simulink model "k64f_rateadapt"  (R2020a)
settings: Solver=FixedStepAuto  StartTime=0.0  StopTime=1.0  FixedStep=1E-3  RelTol=1e-3  EnableMultiTasking=on
undefined symbols (not defined in the file): A0, A1, D0, D1, D10, D11, D12, D13, D2, D3, D4, D5, D6, D7, D8, D9, PTA0, PTA1, PTA2, PTB2, PTB23, PTB3, PTB9, PTC16, PTC17, PTC2, PTC3, PTC4, PTD0, PTD1, PTD2, PTD3
libraries: frdmk64flib x23, etargetslib x2
settings Model: ExtModeTrigDuration=5  Creator=Mostafa  LastModifiedBy=Kevin Chen
settings OptimizationCC: EnhancedBackFolding=on  PassReuseOutputArgsAs=Individual arguments  ZeroExternalMemoryAtStartup=off  ZeroInternalMemoryAtStartup=off  MaxStackSize=64  OptimizeBlockOrder=speed  DifferentSizesBufferReuse=on  OptimizationCustomize=off  EfficientTunableParamExpr=on
settings DebuggingCC: ParameterPrecisionLossMsg=none  ParameterTunabilityLossMsg=error
settings HardwareCC: ProdBitPerPointer=32  ProdBitPerSizeT=32  ProdBitPerPtrDiffT=32  ProdLargestAtomicInteger=Long  ProdLargestAtomicFloat=Double  ProdWordSize=32  ProdHWDeviceType=ARM Compatible->ARM Cortex  UseEmbeddedCoderFeatures=off
settings SFSimCC: MATLABDynamicMemAlloc=off
settings RTWCC: SystemTargetFile=ert.tlc  HardwareBoard=NXP FRDM-K64F  TemplateMakefile=ert_default_tmf  Toolchain=GNU Tools for ARM Embedded Processors
settings CodeAppCC: ForceParamTrailComments=on  IgnoreCustomStorageClasses=off  OperatorAnnotations=on  SimulinkDataObjDesc=on  SFDataObjDesc=on  InsertBlockDesc=on
settings ERTTargetCC: SupportNonInlinedSFcns=on

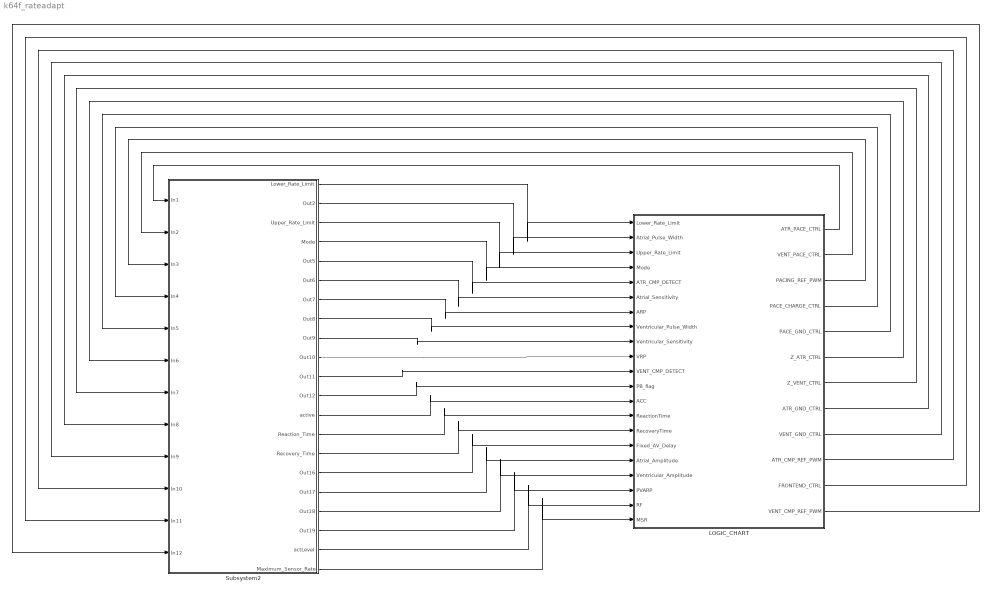
== system k64f_rateadapt ==
  LOGIC_CHART : Stateflow chart  TreatAsAtomicUnit=on
      settings: PortSchema="{\"entries\":[{\"content\":{\"sides\":[{\"content\":{\"connectorIds\":[\"In1\",\"In2\",\"In3\",\"In4\",\"In5\",\"In6\",\"In7\",\"In8\",\"In9\",\"In10\",\"In11\",\"In12\",\"In13\",\"In14\",\"In17\",\"In18\",\"In19\",\"In20\",\"In21\",\"In15\",\"In16\"]},\"type\":\"ConnectorPlacement.EquallySpacedRectSide\",\"uuid\":\"2532a15d-7e3f-497c-8f71-038aa275bfb3\"},{\"content\":{\"connectorIds\":[\"Out1\",\"Out2\",\"Out3\",\"Out4\",\"Out5\",\"Out6\",\"Out7\",\"Out8\",\"Out9\",\"Out10\",\"Out11\",\"Out12\"],\"side\":\"RIGHT\"},\"type\":\"ConnectorPlacement.EquallySpacedRectSide\",\"uuid\":\"b4365400-6566-41c9-a565-c69f74d7ec16\"},{\"content\":{\"connectorIds\":[],\"side\":\"TOP\"},\"type\":\"ConnectorPlacement.EquallySpacedRectSide\",\"uuid\":\"ee6cfb42-5307-4b65-a86e-84b69df89ddc\"}]},\"type\":\"ConnectorPlacement.EquallySpacedConnector\",\"uuid\":\"ec232628-3749-49a9-9e57-0299de21913c\"}],\"packageUris\":[\"http://schema.mathworks.com/mf0/Connector/19700101\"],\"version\":\"1.0\"}"
  Subsystem2 : Subsystem
  wires:
  LOGIC_CHART/1(ATR_PACE_CTRL) -> Subsystem2/1(In1)
  LOGIC_CHART/2(VENT_PACE_CTRL) -> Subsystem2/2(In2)
  LOGIC_CHART/3(PACING_REF_PWM) -> Subsystem2/3(In3)
  LOGIC_CHART/4(PACE_CHARGE_CTRL) -> Subsystem2/4(In4)
  LOGIC_CHART/5(PACE_GND_CTRL) -> Subsystem2/5(In5)
  LOGIC_CHART/6(Z_ATR_CTRL) -> Subsystem2/6(In6)
  LOGIC_CHART/7(Z_VENT_CTRL) -> Subsystem2/7(In7)
  LOGIC_CHART/8(ATR_GND_CTRL) -> Subsystem2/8(In8)
  LOGIC_CHART/9(VENT_GND_CTRL) -> Subsystem2/9(In9)
  LOGIC_CHART/10(ATR_CMP_REF_PWM) -> Subsystem2/10(In10)
  LOGIC_CHART/11(FRONTEND_CTRL) -> Subsystem2/11(In11)
  LOGIC_CHART/12(VENT_CMP_REF_PWM) -> Subsystem2/12(In12)
  Subsystem2/1(Lower_Rate_Limit) -> LOGIC_CHART/1(Lower_Rate_Limit)
  Subsystem2/2(Out2) -> LOGIC_CHART/2(Atrial_Pulse_Width)
  Subsystem2/3(Upper_Rate_Limit) -> LOGIC_CHART/3(Upper_Rate_Limit)
  Subsystem2/4(Mode) -> LOGIC_CHART/4(Mode)
  Subsystem2/5(Out5) -> LOGIC_CHART/5(ATR_CMP_DETECT)
  Subsystem2/6(Out6) -> LOGIC_CHART/6(Atrial_Sensitivity)
  Subsystem2/7(Out7) -> LOGIC_CHART/7(ARP)
  Subsystem2/8(Out8) -> LOGIC_CHART/8(Ventricular_Pulse_Width)
  Subsystem2/9(Out9) -> LOGIC_CHART/9(Ventricular_Sensitivity)
  Subsystem2/10(Out10) -> LOGIC_CHART/10(VRP)
  Subsystem2/11(Out11) -> LOGIC_CHART/11(VENT_CMP_DETECT)
  Subsystem2/12(Out12) -> LOGIC_CHART/12(PB_flag)
  Subsystem2/13(active) -> LOGIC_CHART/13(ACC)
  Subsystem2/14(Reaction_Time) -> LOGIC_CHART/14(ReactionTime)
  Subsystem2/15(Recovery_Time) -> LOGIC_CHART/17(RecoveryTime)
  Subsystem2/16(Out16) -> LOGIC_CHART/18(Fixed_AV_Delay)
  Subsystem2/17(Out17) -> LOGIC_CHART/19(Atrial_Amplitude)
  Subsystem2/18(Out18) -> LOGIC_CHART/20(Ventricular_Amplitude)
  Subsystem2/19(Out19) -> LOGIC_CHART/21(PVARP)
  Subsystem2/20(actLevel) -> LOGIC_CHART/15(RF)
  Subsystem2/21(Maximum_Sensor_Rate) -> LOGIC_CHART/16(MSR)

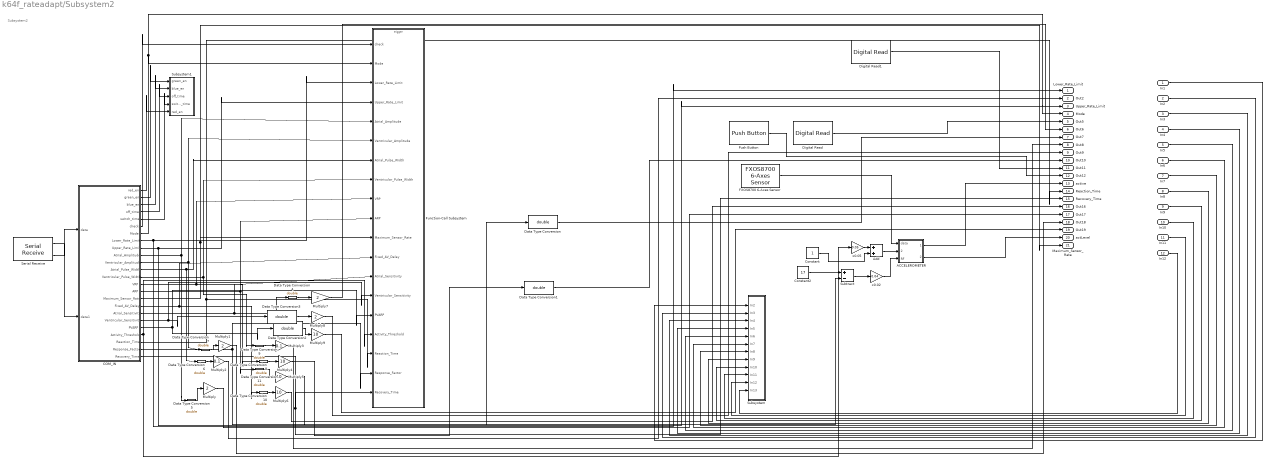
== system k64f_rateadapt/Subsystem2 ==
  note: Subsystem2
  In1 : Inport
  In2 : Inport  Port=2
  In3 : Inport  Port=3
  In4 : Inport  Port=4
  In5 : Inport  Port=5
  In6 : Inport  Port=6
  In7 : Inport  Port=7
  In8 : Inport  Port=8
  In9 : Inport  Port=9
  In10 : Inport  Port=10
  In11 : Inport  Port=11
  In12 : Inport  Port=12
  ACCELEROMETER : Stateflow chart  TreatAsAtomicUnit=on
  Add : Sum
  COM_IN : Stateflow chart  TreatAsAtomicUnit=on
      settings: PortSchema="{\"entries\":[{\"content\":{\"sides\":[{\"content\":{\"connectorIds\":[\"In1\",\"In2\"]},\"type\":\"ConnectorPlacement.EquallySpacedRectSide\",\"uuid\":\"0622ed0d-a63c-4425-81a9-1b700e3d40e7\"},{\"content\":{\"connectorIds\":[\"Out1\",\"Out2\",\"Out3\",\"Out4\",\"Out5\",\"Out24\",\"Out6\",\"Out7\",\"Out8\",\"Out9\",\"Out10\",\"Out11\",\"Out12\",\"Out13\",\"Out14\",\"Out15\",\"Out16\",\"Out17\",\"Out18\",\"Out19\",\"Out20\",\"Out21\",\"Out22\",\"Out23\"],\"side\":\"RIGHT\"},\"type\":\"ConnectorPlacement.EquallySpacedRectSide\",\"uuid\":\"1b9db426-091c-4aed-ac90-de166372e318\"},{\"content\":{\"connectorIds\":[],\"side\":\"TOP\"},\"type\":\"ConnectorPlacement.EquallySpacedRectSide\",\"uuid\":\"c8726b50-1e98-4bba-9c0e-57637e7ead5e\"}]},\"type\":\"ConnectorPlacement.EquallySpacedConnector\",\"uuid\":\"eab4333c-b3ae-429b-bd5d-289e8cbf8e60\"}],\"packageUris\":[\"http://schema.mathworks.com/mf0/Connector/19700101\"],\"version\":\"1.0\"}"
  Constant : Constant
  Constant2 : Constant  Value=17
  Data Type Conversion{,1..11} (12 alike) : DataTypeConversion  OutDataTypeStr=double
  Digital Read : frdmk64flib/Digital Read  Whichpin=PTC16 (D0)  SampleTime=-1
  Digital Read1 : frdmk64flib/Digital Read  Whichpin=PTC17 (D1)  SampleTime=-1
  FXOS8700 6-Axes Sensor : frdmk64flib/FXOS8700 6-Axes Sensor  Activesensor=Accelerometer only  ODR=800Hz  HybridODR=400Hz  Accelfullrange=-4g to +4g  SampleTime=-1
  Function-Call Subsystem : Subsystem  TreatAsAtomicUnit=on
  Multiply{,1,7..8} (4 alike) : Gain  Gain=2
  Multiply2 : Gain  Gain=0.1
  Multiply3 : Gain  Gain=0.1
  Multiply{4..6,9} (4 alike) : Gain  Gain=10
  Push Button : frdmk64flib/Push Button  Whichswitch=SW2  SampleTime1=-1
  Serial Receive : frdmk64flib/Serial Receive  SCIModule=0  Baudrate=uint32(9600)  Parity=None  StopBits=1  HardwareFlowControl=None  ByteOrder=LittleEndian  DataType=uint8  DataLength=20  BlockingMode=off  OutputStatus=on  SampleTime=-1
  Subsystem : Subsystem
  Subsystem1 : Subsystem
  Subtract : Sum  Inputs=+-
  x0.02 : Gain  Gain=0.04
  x0.05 : Gain  Gain=0.05
  Lower_Rate_Limit : Outport
  Out2 : Outport  Port=2
  Upper_Rate_Limit : Outport  Port=3
  Mode : Outport  Port=4
  Out5 : Outport  Port=5
  Out6 : Outport  Port=6
  Out7 : Outport  Port=7
  Out8 : Outport  Port=8
  Out9 : Outport  Port=9
  Out10 : Outport  Port=10
  Out11 : Outport  Port=11
  Out12 : Outport  Port=12
  active : Outport  Port=13
  Reaction_Time : Outport  Port=14
  Recovery_Time : Outport  Port=15
  Out16 : Outport  Port=16
  Out17 : Outport  Port=17
  Out18 : Outport  Port=18
  Out19 : Outport  Port=19
  actLevel : Outport  Port=20
  Maximum_Sensor_Rate : Outport  Port=21
  wires:
  Data Type Conversion5/1 -> Multiply/1
  In11/1 -> Subsystem/11(In12)
  COM_IN/2(green_en) -> Subsystem1/1(green_en)
  FXOS8700 6-Axes Sensor/1 -> ACCELEROMETER/1(data)
  ACCELEROMETER/1(active) -> active/1
  COM_IN/10(Ventricular_Amplitude) -> Data Type Conversion7/1, Function-Call Subsystem/6(Ventricular_Amplitude)
  COM_IN/7(Lower_Rate_Limit) -> Lower_Rate_Limit/1, Function-Call Subsystem/3(Lower_Rate_Limit)
  x0.02/1 -> ACCELEROMETER/3(RF)
  COM_IN/20(Activity_Threshold) -> x0.05/1, Function-Call Subsystem/16(Activity_Threshold)
  Data Type Conversion9/1 -> Multiply3/1
  Serial Receive/1 -> COM_IN/2(data1)
  COM_IN/12(Ventricular_Pulse_Width) -> Data Type Conversion9/1, Function-Call Subsystem/8(Ventricular_Pulse_Width)
  COM_IN/11(Atrial_Pulse_Width) -> Function-Call Subsystem/7(Atrial_Pulse_Width), Data Type Conversion6/1
  Add/1 -> ACCELEROMETER/2(Threshold)
  Data Type Conversion4/1 -> Multiply7/1
  COM_IN/18(Ventricular_Sensitivity) -> Data Type Conversion3/1, Function-Call Subsystem/14(Ventricular_Sensitivity)
  COM_IN/17(Atrial_Sensitivity) -> Data Type Conversion4/1, Function-Call Subsystem/13(Atrial_Sensitivity)
  COM_IN/15(Maximum_Sensor_Rate) -> Maximum_Sensor_Rate/1, Function-Call Subsystem/11(Maximum_Sensor_Rate)
  COM_IN/16(Fixed_AV_Delay) -> Data Type Conversion10/1, Function-Call Subsystem/12(Fixed_AV_Delay)
  COM_IN/6(Mode) -> Mode/1, Function-Call Subsystem/2(Mode)
  Data Type Conversion2/1 -> Multiply9/1
  In4/1 -> Subsystem/4(In5)
  Data Type Conversion3/1 -> Multiply8/1
  Data Type Conversion/1 -> Out7/1
  Data Type Conversion7/1 -> Multiply1/1
  In8/1 -> Subsystem/8(In9)
  Data Type Conversion11/1 -> Multiply5/1
  In6/1 -> Subsystem/6(In7)
  Multiply1/1 -> Out18/1
  COM_IN/21(Reaction_Time) -> Reaction_Time/1, Function-Call Subsystem/17(Reaction_Time)
  Multiply9/1 -> Out19/1
  x0.05/1 -> Add/1
  Constant2/1 -> Subtract/1
  In1/1 -> Subsystem/1(In2)
  Constant/1 -> Add/2
  COM_IN/4(off_time) -> Subsystem1/3(off_time)
  In7/1 -> Subsystem/7(In8)
  COM_IN/9(Atrial_Amplitude) -> Data Type Conversion5/1, Function-Call Subsystem/5(Atrial_Amplitude)
  Data Type Conversion10/1 -> Multiply6/1
  Subtract/1 -> x0.02/1
  COM_IN/13(VRP) -> Data Type Conversion8/1, Function-Call Subsystem/9(VRP)
  Data Type Conversion1/1 -> Out10/1
  COM_IN/19(PVARP) -> Data Type Conversion2/1, Function-Call Subsystem/15(PVARP)
  COM_IN/8(Upper_Rate_Limit) -> Upper_Rate_Limit/1, Function-Call Subsystem/4(Upper_Rate_Limit)
  COM_IN/24(check) -> Function-Call Subsystem/1(check)
  COM_IN/22(Response_Factor) -> Subtract/2, Function-Call Subsystem/18(Response_Factor)
  Digital Read1/1 -> Out11/1
  COM_IN/23(Recovery_Time) -> Recovery_Time/1, Function-Call Subsystem/19(Recovery_Time)
  COM_IN/14(ARP) -> Data Type Conversion11/1, Function-Call Subsystem/10(ARP)
  Data Type Conversion6/1 -> Multiply2/1
  Push Button/1 -> Out12/1
  Multiply4/1 -> Data Type Conversion1/1
  Serial Receive/2 -> COM_IN/1(data)
  COM_IN/5(switch_time) -> Subsystem1/4(switch_time)
  In2/1 -> Subsystem/2(In3)
  COM_IN/3(blue_en) -> Subsystem1/2(blue_en)
  COM_IN/1(red_en) -> Subsystem1/5(red_en)
  Multiply5/1 -> Data Type Conversion/1
  ACCELEROMETER/2(actLevel) -> actLevel/1
  Data Type Conversion8/1 -> Multiply4/1
  In3/1 -> Subsystem/3(In4)
  In9/1 -> Subsystem/9(In10)
  Digital Read/1 -> Out5/1
  In5/1 -> Subsystem/5(In6)
  In12/1 -> Subsystem/12(In13)
  In10/1 -> Subsystem/10(In11)
  Multiply7/1 -> Out6/1
  Multiply6/1 -> Out16/1
  Multiply8/1 -> Out9/1
  Multiply2/1 -> Out2/1
  Multiply3/1 -> Out8/1
  Multiply/1 -> Out17/1

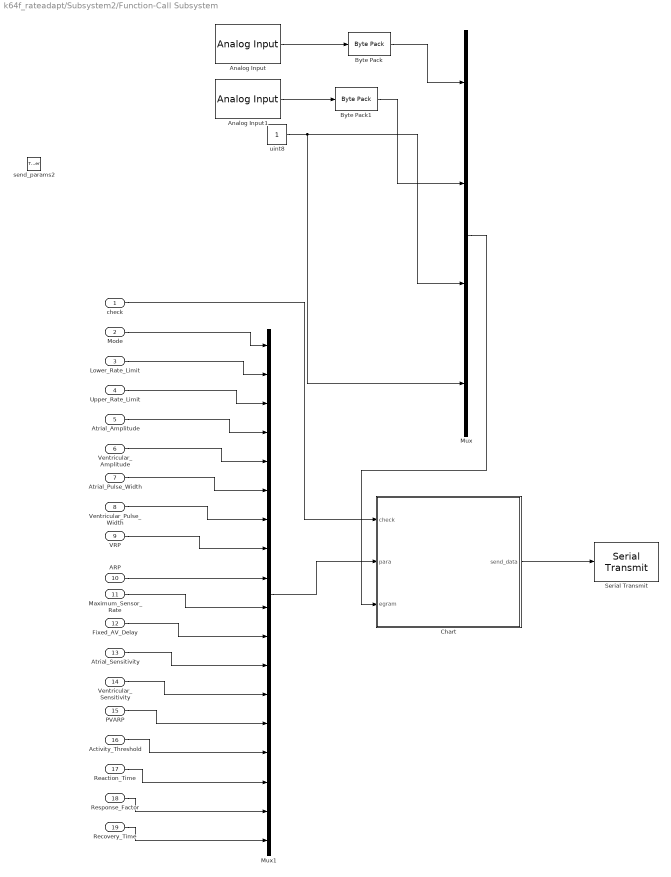
== system k64f_rateadapt/Subsystem2/Function-Call Subsystem ==
  check : Inport
  Mode : Inport  Port=2
  Lower_Rate_Limit : Inport  Port=3
  Upper_Rate_Limit : Inport  Port=4
  Atrial_Amplitude : Inport  Port=5
  Ventricular_Amplitude : Inport  Port=6
  Atrial_Pulse_Width : Inport  Port=7
  Ventricular_Pulse_Width : Inport  Port=8
  VRP : Inport  Port=9
  ARP : Inport  Port=10
  Maximum_Sensor_Rate : Inport  Port=11
  Fixed_AV_Delay : Inport  Port=12
  Atrial_Sensitivity : Inport  Port=13
  Ventricular_Sensitivity : Inport  Port=14
  PVARP : Inport  Port=15
  Activity_Threshold : Inport  Port=16
  Reaction_Time : Inport  Port=17
  Response_Factor : Inport  Port=18
  Recovery_Time : Inport  Port=19
  send_params2 : TriggerPort  TriggerType=function-call  IsSimulinkFunction=on  FunctionName=send_params2  VariantControl=Variant
  Analog Input : frdmk64flib/Analog Input  Whichpin=PTB2 (A0)  SampleTime=-1
  Analog Input1 : frdmk64flib/Analog Input  Whichpin=PTB3 (A1)  SampleTime=-1
  Byte Pack : etargetslib/Byte Pack  datatypes={'double'}  byteAlign=1
  Byte Pack1 : etargetslib/Byte Pack  datatypes={'double'}  byteAlign=1
  Chart : Stateflow chart  TreatAsAtomicUnit=on
  Mux : Mux
  Mux1 : Mux  Inputs=18
  Serial Transmit : frdmk64flib/Serial Transmit  SCIModule=0  Baudrate=uint32(9600)  Parity=None  StopBits=1  HardwareFlowControl=None  ByteOrder=LittleEndian  BlockingMode=on  OutputStatus=off
  uint8 : Constant  OutDataTypeStr=uint8
  wires:
  Mode/1 -> Mux1/1
  check/1 -> Chart/1(check)
  Analog Input1/1 -> Byte Pack1/1
  Chart/1(send_data) -> Serial Transmit/1
  Lower_Rate_Limit/1 -> Mux1/2
  Mux1/1 -> Chart/2(para)
  Upper_Rate_Limit/1 -> Mux1/3
  Mux/1 -> Chart/3(egram)
  Atrial_Amplitude/1 -> Mux1/4
  uint8/1 -> Mux/4, Mux/3
  Analog Input/1 -> Byte Pack/1
  Byte Pack/1 -> Mux/1
  Byte Pack1/1 -> Mux/2
  Ventricular_Amplitude/1 -> Mux1/5
  Atrial_Pulse_Width/1 -> Mux1/6
  Ventricular_Pulse_Width/1 -> Mux1/7
  VRP/1 -> Mux1/8
  Maximum_Sensor_Rate/1 -> Mux1/10
  Fixed_AV_Delay/1 -> Mux1/11
  Atrial_Sensitivity/1 -> Mux1/12
  Ventricular_Sensitivity/1 -> Mux1/13
  PVARP/1 -> Mux1/14
  Reaction_Time/1 -> Mux1/16
  Activity_Threshold/1 -> Mux1/15
  Response_Factor/1 -> Mux1/17
  Recovery_Time/1 -> Mux1/18
  ARP/1 -> Mux1/9

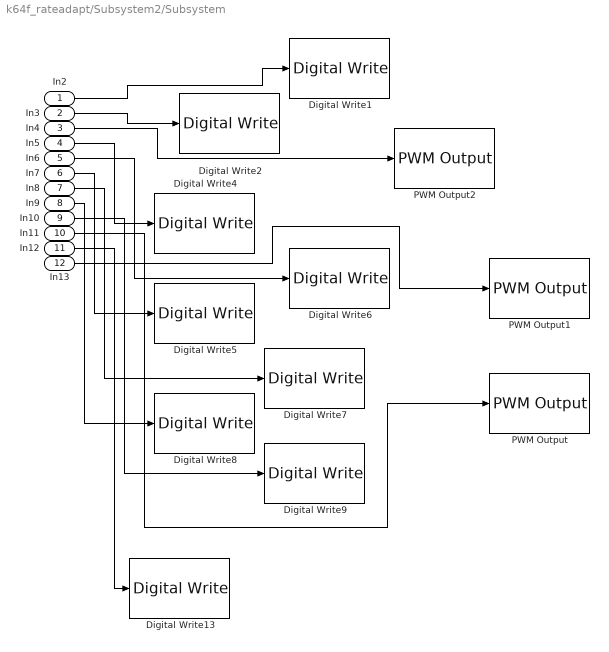
== system k64f_rateadapt/Subsystem2/Subsystem ==
  In2 : Inport
  In3 : Inport  Port=2
  In4 : Inport  Port=3
  In5 : Inport  Port=4
  In6 : Inport  Port=5
  In7 : Inport  Port=6
  In8 : Inport  Port=7
  In9 : Inport  Port=8
  In10 : Inport  Port=9
  In11 : Inport  Port=10
  In12 : Inport  Port=11
  In13 : Inport  Port=12
  Digital Write1 : frdmk64flib/Digital Write  Whichpin=PTA0 (D8)
  Digital Write13 : frdmk64flib/Digital Write  Whichpin=PTD1 (D13)
  Digital Write2 : frdmk64flib/Digital Write  Whichpin=PTC4 (D9)
  Digital Write4 : frdmk64flib/Digital Write  Whichpin=PTB9 (D2)
  Digital Write5 : frdmk64flib/Digital Write  Whichpin=PTB23 (D4)
  Digital Write6 : frdmk64flib/Digital Write  Whichpin=PTD0 (D10)
  Digital Write7 : frdmk64flib/Digital Write  Whichpin=PTC3 (D7)
  Digital Write8 : frdmk64flib/Digital Write  Whichpin=PTD2 (D11)
  Digital Write9 : frdmk64flib/Digital Write  Whichpin=PTD3 (D12)
  PWM Output : frdmk64flib/PWM Output  Whichpin=PTC2 (D6)  InitialFrequency=2000  InitialDutyCycle=100
  PWM Output1 : frdmk64flib/PWM Output  Whichpin=PTA1 (D3)  InitialFrequency=2000  InitialDutyCycle=0
  PWM Output2 : frdmk64flib/PWM Output  Whichpin=PTA2 (D5)  InitialFrequency=2000  InitialDutyCycle=100
  wires:
  In5/1 -> Digital Write4/1
  In9/1 -> Digital Write8/1
  In7/1 -> Digital Write5/1
  In3/1 -> Digital Write2/1
  In6/1 -> Digital Write6/1
  In4/1 -> PWM Output2/1
  In8/1 -> Digital Write7/1
  In10/1 -> Digital Write9/1
  In2/1 -> Digital Write1/1
  In12/1 -> Digital Write13/1
  In11/1 -> PWM Output/1
  In13/1 -> PWM Output1/1

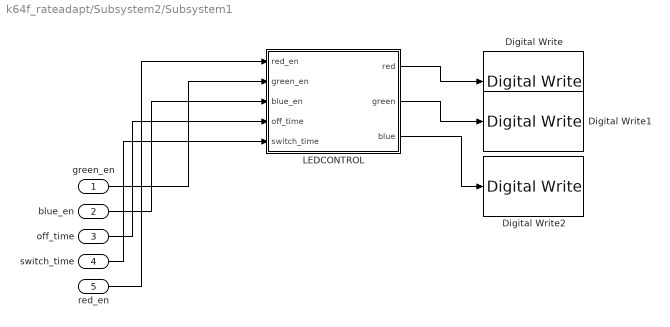
== system k64f_rateadapt/Subsystem2/Subsystem1 ==
  green_en : Inport
  blue_en : Inport  Port=2
  off_time : Inport  Port=3
  switch_time : Inport  Port=4
  red_en : Inport  Port=5
  Digital Write : frdmk64flib/Digital Write  Whichpin=RED_LED
  Digital Write1 : frdmk64flib/Digital Write  Whichpin=GREEN_LED
  Digital Write2 : frdmk64flib/Digital Write  Whichpin=BLUE_LED
  LEDCONTROL : Stateflow chart  TreatAsAtomicUnit=on
  wires:
  LEDCONTROL/1(red) -> Digital Write/1
  green_en/1 -> LEDCONTROL/2(green_en)
  LEDCONTROL/3(blue) -> Digital Write2/1
  switch_time/1 -> LEDCONTROL/5(switch_time)
  LEDCONTROL/2(green) -> Digital Write1/1
  red_en/1 -> LEDCONTROL/1(red_en)
  blue_en/1 -> LEDCONTROL/3(blue_en)
  off_time/1 -> LEDCONTROL/4(off_time)

== stateflow chart k64f_rateadapt/Subsystem2/COM_IN ==
  settings: executeAtInitialization=1
  state AOO
    entry:
    Mode=data1(3);
    Lower_Rate_Limit = data1(4);
    Upper_Rate_Limit = data1(5);
    Atrial_Amplitude = data1(6);
    Ventricular_Amplitude =data1(7);
    Atrial_Pulse_Width = data1(8);
    Ventricular_Pulse_Width = data1(9);
    VRP = data1(10);
    ARP = data1(11);
    Maximum_Sensor_Rate = data1(12);
    Fixed_AV_Delay = data1(13);
    Atrial_Sensitivity = data1(14);
    Ventricular_Sensitivity =data1(15);
    PVARP = data1(16);
    Activity_Threshold = data1(17);
    Reaction_Time = data1(18);
    Response_Factor = data1(19);
    Recovery_Time = data1(20);
    blue_en=0;
    red_en=0;
    green_en=1;
  state Idle
    entry:
    red_en=1;
    green_en=0;
    blue_en=0;
    off_time=0.5;
    switch_time=200;
  state Standby
    entry:
    red_en=0;
    blue_en=1;
    green_en=0;
    check=0;
  state ECHO_PARAM
    entry:
    check=49;
    send_params2();
    blue_en=0;
    red_en=1;
  state ECHO_EGRAM
    entry:
    check=47;
    send_params2();
    blue_en=1;
    green_en=1;
  (default) -> Idle
  AOO -> Standby : [after(2,sec)]
  (junction 205) -> AOO [order 1] : [data1(2)==hex2dec("55")]
  Idle -> Standby
  (junction 205) -> ECHO_EGRAM [order 3] : [data1(2)==hex2dec("47")]
  (junction 214) -> (junction 205) : [data1(1)==hex2dec("16")]
  (junction 205) -> ECHO_PARAM [order 2] : [data1(2)==hex2dec("49")]
  ECHO_EGRAM -> Standby [order 1] : [data1(2)==hex2dec("62")]
  Standby -> (junction 214) : [data==0]
  ECHO_PARAM -> Standby : [after(2,sec)]
  ECHO_EGRAM -> ECHO_EGRAM [order 2] : [after(1,msec)]
  data: data input uint8; data1 input uint8; red_en output uint8; green_en output uint8; blue_en output 'uint8'; off_time output 'single'; switch_time output 'uint16'; Mode output; Lower_Rate_Limit output; Upper_Rate_Limit output; Atrial_Amplitude output; Ventricular_Amplitude output; Atrial_Pulse_Width output; Ventricular_Pulse_Width output; VRP output; ARP output; Maximum_Sensor_Rate output; Fixed_AV_Delay output; Atrial_Sensitivity output; Ventricular_Sensitivity output; PVARP output; Activity_Threshold output; Reaction_Time output; Response_Factor output; Recovery_Time output; check output

== stateflow chart k64f_rateadapt/Subsystem2/ACCELEROMETER ==
  state Enter
    entry:
    active=0;
    actLevel=0;
  state Ini
    entry:
    Timing=0;
    acc=0;
  state H
    entry:
    acc=acc+norm(data);
    %update the motion level every 0.5s
    if(Timing==500)
    acc=acc/100; %taking average of acc over 0.5s
    if(acc>Threshold)
    active=1;
    if((acc-Threshold)>=RF)
    actLevel=100; %MSR will be reached if actLevel=100
    else
    %actLevel is the proportion of acc above threshold, in percentage
    actLevel=(acc-Threshold)/RF*100;
    end
    else %if acc is below threshold
    active=0;
    actLevel=0;
    end
    end
  (default) -> Enter
  Enter -> Ini
  Ini -> H
  H -> Ini [order 2] : [Timing>=500]
  H -> H [order 1] : [after(5,msec)&&Timing<500]{Timing=Timing+5}
      | %accumulate new motion data every 5ms
  data: data input; active output; actLevel output; acc local; Timing local; Threshold input; RF input

== stateflow chart k64f_rateadapt/LOGIC_CHART ==
  state VOO_CHARGING
    entry:
    %parameters for charging c22
    ATR_PACE_CTRL= false;
    VENT_PACE_CTRL = false;
    PACING_REF_PWM = Ventricular_Amplitude;
    PACE_CHARGE_CTRL = true;
    %parameters for discharging into c11
    PACE_GND_CTRL = true;
    VENT_PACE_CTRL = false;
    Z_ATR_CTRL = false;
    Z_VENT_CTRL = false;
    ATR_PACE_CTRL= false;
    ATR_GND_CTRL = false;
    VENT_GND_CTRL = true;
    if(Mode==9) %if it's rate adaptive
    if(ACC==1) %if activity above threshold
    %if rate is lower than the expected rate at the detected activity level
    %RF is the actLevel from Accelerometer FSM, which
    % is the proportion of acc above threshold, in percentage
    if((Rate-Lower_Rate_Limit)<((MSR-Lower_Rate_Limit)*RF/100))
    %increase Rate at the rate required to reach MSR from LRL within reaction time
    Rate=(Rate+(MSR-Lower_Rate_Limit)/ReactionTime*60/Rate);
    else
    %rate stays at the expected rate, determined from the current MSR, LRL and RF
    Rate=((MSR-Lower_Rate_Limit)*RF/100+Lower_Rate_Limit);
    end
    else %Acc==0, below threshold
    if(Rate>Lower_Rate_Limit)
    %decrease Rate at the rate required to reach MSR from LRL within recovery time
    Rate=(Rate-(MSR-Lower_Rate_Limit)/RecoveryTime*60/Rate);
    else
    Rate=Lower_Rate_Limit;
    end
    end
    end
  state DELAY_STATE3
    %delay for bonus
  state VOO_PACING
    entry:
    PACE_CHARGE_CTRL = false;
    PACE_GND_CTRL = true;
    ATR_PACE_CTRL= false;
    ATR_GND_CTRL = false;
    Z_ATR_CTRL = false;
    Z_VENT_CTRL = false;
    VENT_GND_CTRL = false;
    VENT_PACE_CTRL = true;
  state DELAY_STATE
    %delay for bonus
  state AOO_CHARGING
    entry:
    %parameters for charging c22
    ATR_PACE_CTRL= false;
    VENT_PACE_CTRL = false;
    PACING_REF_PWM =  Atrial_Amplitude;
    PACE_CHARGE_CTRL = true;
    %parameters for discharging into c11
    PACE_GND_CTRL = true;
    VENT_PACE_CTRL = false;
    Z_ATR_CTRL = false;
    Z_VENT_CTRL = false;
    ATR_PACE_CTRL= false;
    ATR_GND_CTRL = true;
    VENT_GND_CTRL = false;
    if(Mode==7) %if it's rate adaptive
    %for detailed comments of the following part of code, refer to VOO(R) mode
    if(ACC==1)
    if((Rate-Lower_Rate_Limit)<((MSR-Lower_Rate_Limit)*RF/100))
    Rate=(Rate+(MSR-Lower_Rate_Limit)/ReactionTime*60/Rate);
    else
    Rate=((MSR-Lower_Rate_Limit)*RF/100+Lower_Rate_Limit);
    end
    else
    if(Rate>Lower_Rate_Limit)
    Rate=(Rate-(MSR-Lower_Rate_Limit)/RecoveryTime*60/Rate);
    else
    Rate=Lower_Rate_Limit;
    end
    end
    end
  state AOO_PACING
    entry:
    PACE_CHARGE_CTRL = false;
    PACE_GND_CTRL = true;
    ATR_PACE_CTRL= true;
    ATR_GND_CTRL = false;
    Z_ATR_CTRL = false;
    Z_VENT_CTRL = false;
    VENT_GND_CTRL = false;
    VENT_PACE_CTRL = false;
  state Initial
    entry:
    delay=0;
    Rate=Lower_Rate_Limit;
    %delay is used in AAI(R)&VVI(R)
    %to correct for delay caused
    %by ARP and VRP
    %Rate is fixed to LRL if it's not in rate adaptive
    %modes, and it's changeable
    %if used in rate adaptive modes
  state AAI_CHARGING
    entry:
    %parameters for charging c22
    ATR_PACE_CTRL= false;
    VENT_PACE_CTRL = false;
    PACING_REF_PWM =  Atrial_Amplitude;
    PACE_CHARGE_CTRL = true;
    %parameters for discharging into c11
    PACE_GND_CTRL = true;
    VENT_PACE_CTRL = false;
    Z_ATR_CTRL = false;
    Z_VENT_CTRL = false;
    ATR_PACE_CTRL= false;
    ATR_GND_CTRL = true;
    VENT_GND_CTRL = false;
    %parameters for sensing
    ATR_CMP_REF_PWM=Atrial_Sensitivity;
    FRONTEND_CTRL= true;
    %timing for an expected natural heart event
    Timing=int16(0);
    if(Mode==8) %if it's rate adaptive
    %for detailed comments of the following part of code, refer to VOO(R) mode
    if(ACC==1)
    if((Rate-Lower_Rate_Limit)<((MSR-Lower_Rate_Limit)*RF/100))
    Rate=(Rate+(MSR-Lower_Rate_Limit)/ReactionTime*60/Rate);
    else
    Rate=((MSR-Lower_Rate_Limit)*RF/100+Lower_Rate_Limit);
    end
    else
    if(Rate>Lower_Rate_Limit)
    Rate=(Rate-(MSR-Lower_Rate_Limit)/RecoveryTime*60/Rate);
    else
    Rate=Lower_Rate_Limit;
    end
    end
    end
  state AAI_PACING
    entry:
    PACE_CHARGE_CTRL = false;
    PACE_GND_CTRL = true;
    ATR_PACE_CTRL= true;
    ATR_GND_CTRL = false;
    Z_ATR_CTRL = false;
    Z_VENT_CTRL = false;
    VENT_GND_CTRL = false;
    VENT_PACE_CTRL = false;
  state DOO_CHARGE1
    entry:
    FRONTEND_CTRL = false;
    PACE_GND_CTRL = true;
    VENT_PACE_CTRL = true;
    Z_ATR_CTRL = false;
    Z_VENT_CTRL = false;
    ATR_GND_CTRL = true;
    VENT_GND_CTRL = true;
    ATR_PACE_CTRL=false;
    VENT_PACE_CTRL=false;
    PACE_CHARGE_CTRL=true;
    PACING_REF_PWM = Ventricular_Amplitude;
    if(Mode==6) %if it's rate adaptive
    %for detailed comments of the following part of code, refer to VOO(R) mode
    if(ACC==1)
    if((Rate-Lower_Rate_Limit)<((MSR-Lower_Rate_Limit)*RF/100))
    Rate=(Rate+(MSR-Lower_Rate_Limit)/ReactionTime*60/Rate);
    else
    Rate=((MSR-Lower_Rate_Limit)*RF/100+Lower_Rate_Limit);
    end
    else
    if(Rate>Lower_Rate_Limit)
    Rate=(Rate-(MSR-Lower_Rate_Limit)/RecoveryTime*60/Rate);
    else
    Rate=Lower_Rate_Limit;
    end
    end
    end
  state AV_PACING2
    entry: %atrial pacing
    PACE_CHARGE_CTRL=false;
    ATR_GND_CTRL=false;
    VENT_GND_CTRL=false;
    PACE_GND_CTRL=true;
    VENT_PACE_CTRL=false;
    ATR_PACE_CTRL=true;
  state DELAY_STATE2
    %delay for bonus
  state AV_Delay2
    entry:
    ATR_PACE_CTRL=false;
    %av delay
  state VVI_CHARGING
    entry:
    %parameters for charging c22
    ATR_PACE_CTRL= false;
    VENT_PACE_CTRL = false;
    PACING_REF_PWM =  Ventricular_Amplitude;
    PACE_CHARGE_CTRL = true;
    %parameters for discharging into c11
    PACE_GND_CTRL = true;
    VENT_PACE_CTRL = false;
    Z_ATR_CTRL = false;
    Z_VENT_CTRL = false;
    ATR_PACE_CTRL= false;
    ATR_GND_CTRL = false;
    VENT_GND_CTRL = true;
    %sensing
    VENT_CMP_REF_PWM=Ventricular_Sensitivity;
    FRONTEND_CTRL= true;
    %timing for an expected natural heart event
    Timing=int16(0);
    if(Mode==10) %if it's rate adaptive
    %for detailed comments of the following part of code, refer to VOO(R) mode
    if(ACC==1)
    if((Rate-Lower_Rate_Limit)<((MSR-Lower_Rate_Limit)*RF/100))
    Rate=(Rate+(MSR-Lower_Rate_Limit)/ReactionTime*60/Rate);
    else
    Rate=((MSR-Lower_Rate_Limit)*RF/100+Lower_Rate_Limit);
    end
    else
    if(Rate>Lower_Rate_Limit)
    Rate=(Rate-(MSR-Lower_Rate_Limit)/RecoveryTime*60/Rate);
    else
    Rate=Lower_Rate_Limit;
    end
    end
    end
  state VV_PACING2
    entry: %pacing ventricle
    PACE_CHARGE_CTRL=false;
    ATR_GND_CTRL=false;
    VENT_GND_CTRL=false;
    PACE_GND_CTRL=true;
    ATR_PACE_CTRL=false;
    VENT_PACE_CTRL=true;
  state DELAY_STATE4
    %delay for bonus
  state AAI_SENSING
    entry:
    ATR_CMP_REF_PWM=Atrial_Sensitivity;
    FRONTEND_CTRL= true;
    Detect=ATR_CMP_DETECT;
  state VVI_PACING
    entry:
    PACE_CHARGE_CTRL = false;
    PACE_GND_CTRL = true;
    ATR_PACE_CTRL= false;
    ATR_GND_CTRL = false;
    Z_ATR_CTRL = false;
    Z_VENT_CTRL = false;
    VENT_GND_CTRL = false;
    VENT_PACE_CTRL = true;
  state DELAY_STATE1
    %delay for bonus
  state VVI_SENSING
    entry:
    VENT_CMP_REF_PWM=Ventricular_Sensitivity;
    FRONTEND_CTRL= true;
    Detect=VENT_CMP_DETECT;
  DELAY_STATE3 -> VOO_CHARGING : [PB_flag == 0]
  VOO_CHARGING -> DELAY_STATE3 [order 2] : [PB_flag == 1]
  VOO_CHARGING -> VOO_PACING [order 1] : [after(60000/Rate-Ventricular_Pulse_Width, msec)]
  VOO_PACING -> VOO_CHARGING : [after(Ventricular_Pulse_Width, msec)]
  Initial -> VOO_CHARGING [order 2] : [Mode==4 || Mode==9] %VOO(R)
  DELAY_STATE -> AOO_CHARGING : [PB_flag == 0]
  VOO_CHARGING -> Initial [order 3] : [Mode~=4&&Mode~=9]
  AOO_CHARGING -> DELAY_STATE [order 2] : [PB_flag == 1]
  AOO_CHARGING -> AOO_PACING [order 1] : [after(60000/Rate-Atrial_Pulse_Width, msec)]
  AOO_PACING -> AOO_CHARGING : [after(Atrial_Pulse_Width, msec)]
  Initial -> AOO_CHARGING [order 1] : [Mode==2||Mode==7]%AOO(R)
  (default) -> Initial
  AOO_CHARGING -> Initial [order 3] : [Mode~=2&&Mode~=7]
  AAI_CHARGING -> Initial [order 3] : [Mode~=3&&Mode~=8]
  Initial -> AAI_CHARGING [order 5] : [Mode==3||Mode==8]%AAI(R)
  Initial -> DOO_CHARGE1 [order 3] : [Mode ==1||Mode==6]%DOO(R)
  DOO_CHARGE1 -> Initial [order 2] : [Mode~=1&&Mode~=6]%if mode has been switched
  VVI_CHARGING -> Initial [order 3] : [Mode~=5&&Mode~=10]
  Initial -> VVI_CHARGING [order 4] : [Mode==5||Mode==10] %VVI(R)
  DOO_CHARGE1 -> AV_PACING2 [order 1] : after(60000/Rate-Atrial_Pulse_Width-Fixed_AV_Delay-Ventricular_Pulse_Width,msec)
  AAI_PACING -> AAI_CHARGING : [after(Atrial_Pulse_Width, msec)]{delay=0;}
  AAI_SENSING -> AAI_PACING [order 2] : [after (1, msec) && Detect==false && Timing>=int16(60000/Rate-Atrial_Pulse_Width-delay)]%timeout. A pacing occurs
  DELAY_STATE2 -> AAI_CHARGING : [PB_flag == 0]
  AAI_CHARGING -> DELAY_STATE2 [order 2] : [PB_flag == 1]
  AV_PACING2 -> AV_Delay2 : after(Atrial_Pulse_Width,msec)
  AV_Delay2 -> VV_PACING2 : after(Fixed_AV_Delay,msec)
  DELAY_STATE4 -> DOO_CHARGE1 : [PB_flag == 0]
  (junction 165) -> AAI_CHARGING : [after(ARP, msec)]{delay=ARP;} %set delay to compensate for ARP
  AAI_SENSING -> (junction 165) [order 3] : [after (1, msec) && Detect==true]%if a natural event detected
  AAI_CHARGING -> AAI_SENSING [order 1] : [PB_flag==0]
  DOO_CHARGE1 -> DELAY_STATE4 [order 3] : [PB_flag == 1]
  VV_PACING2 -> DOO_CHARGE1 : after(Ventricular_Pulse_Width,msec)
  AAI_SENSING -> AAI_SENSING [order 1] : [after (1, msec) && Detect==false && Timing<int16(60000/Rate-Atrial_Pulse_Width-delay)]{Timing = Timing +1}%senses every 1ms, and timing counts up by 1
  DELAY_STATE1 -> VVI_CHARGING : [PB_flag == 0]
  VVI_PACING -> VVI_CHARGING : [after(Ventricular_Pulse_Width, msec)]{delay=0;}
  VVI_CHARGING -> DELAY_STATE1 [order 2] : [PB_flag == 1]
  VVI_CHARGING -> VVI_SENSING [order 1] : [PB_flag==0]
  (junction 204) -> VVI_CHARGING : [after(VRP, msec)]{delay=VRP;}%set delay to compensate for VRP
  VVI_SENSING -> VVI_PACING [order 2] : [after (1, msec) && Detect==false && Timing>=int16(60000/Rate-Ventricular_Pulse_Width-delay)]
      | %timeout. A pacing occurs
  VVI_SENSING -> (junction 204) [order 3] : [after(1,msec)&&Detect==true] %if a natural event detected
  VVI_SENSING -> VVI_SENSING [order 1] : [after (1, msec) && Detect==false && Timing<int16(60000/Rate-Ventricular_Pulse_Width-delay)]{Timing = Timing +1;}%senses every 1ms, and timing counts up by 1
  data: ATR_PACE_CTRL output; VENT_PACE_CTRL output; PACING_REF_PWM output; PACE_CHARGE_CTRL output; PACE_GND_CTRL output; Z_ATR_CTRL output; Z_VENT_CTRL output; ATR_GND_CTRL output; VENT_GND_CTRL output; Lower_Rate_Limit input; Atrial_Pulse_Width input; Upper_Rate_Limit input; Mode input; ATR_CMP_DETECT input; ATR_CMP_REF_PWM output; Atrial_Sensitivity input; ARP input; FRONTEND_CTRL output; Timing local; GREEN_LED constant double; Detect local; Ventricular_Pulse_Width input; Ventricular_Sensitivity input; VRP input; VENT_CMP_DETECT input; VENT_CMP_REF_PWM output; PB_flag input; ACC input; ReactionTime input; Rate local; RF input; MSR input; RecoveryTime input; delay local; Fixed_AV_Delay input; Atrial_Amplitude input; Ventricular_Amplitude input; PVARP input

== stateflow chart k64f_rateadapt/Subsystem2/Function-Call Subsystem/Chart ==
  state SEND_PARA
    entry:
    send_data=para;
  state IN
  state SEND_EGRAM
    entry:
    send_data=egram;
  SEND_PARA -> IN
  IN -> SEND_PARA [order 2] : [check==49]
  (default) -> IN
  SEND_EGRAM -> IN
  IN -> SEND_EGRAM [order 1] : [check==47]
  data: check input; send_data output; para input; egram input

== stateflow chart k64f_rateadapt/Subsystem2/Subsystem1/LEDCONTROL ==
  state OFF
    entry:
    red=0;
    green=0;
    blue=0;
  state RED_ON
    entry:
    red=1;
    green=0;
    blue=0;
  state BLUE_ON
    entry:
    red=0;
    green=0;
    blue=1;
  state GREEN_ON
    entry:
    red=0;
    green=1;
    blue=0;
  (default) -> OFF
  OFF -> (junction 20) : [after(off_time,sec)]
  (junction 20) -> RED_ON [order 1] : [red_en==1]
  (junction 20) -> (junction 10) [order 2]
  (junction 16) -> OFF
  RED_ON -> (junction 10) : [after(switch_time,msec)]
  (junction 10) -> (junction 12) [order 2]
  (junction 10) -> GREEN_ON [order 1] : [green_en==1]
  (junction 12) -> (junction 16) [order 2]
  BLUE_ON -> (junction 16) : [after(switch_time,msec)]
  (junction 12) -> BLUE_ON [order 1] : [blue_en==1]
  GREEN_ON -> (junction 12) : [after(switch_time,msec)]
  data: red_en input; green_en input; blue_en input; off_time input; switch_time input; red output; green output; blue output
